simulink model "IEEE123_4subsystem"  (R2022b)
settings: Solver=ode4  StartTime=0.0  StopTime=inf  FixedStep=Ts  MaxStep=1e-4  RelTol=1e-3
PreLoadFcn:
  | Ts = 50e-6;
PostLoadFcn:
  | Ts = 50e-6;
InitFcn:
  | %%%%%%%%%%%%%%%%%%%%%%%%
  | % Simulation data for the IEEE 123 Node Test Feeder model
  | %%%%%%%%%%%%%%%%%%%%%%%
  | 
  | % miles/km
  | mi2km = 1.60934;
  | 
  | % feet to km
  | ft2km = 0.0003048;
  | 
  | % microsiemens to Farads
  | ms2F = 1/2/pi/60*1e-6;
  | 
  | %% Configuration 1 - series reactance - ohm/mile
  | 
  | R_1 = [0.4576 0.1560 0.1535;0.1560 0.4666 0.1580;0.1535 0.1580 0.4615];
  | X_1 = [1.0780 0.5017 0.3849;0.5017 1.0482 0.4236;0.3849 0.4236 1.0651];
  | 
  | % charging susceptance - microsiemens/mile
  | 
  | B_1 = [5.6765 -1.8319 -0.6982;-1.8319 5.9809 -1.1645;-0.6982 -1.1645 5.3971];
  | 
  | % convert for SPS
  | 
  | R_1 = R_1/mi2km;
  | 
  | Rs_1=(R_1(1,1)+R_1(2,2)+R_1(3,3))/3;
  | Rm_1=(R_1(1,2)+R_1(1,3)+R_1(2,3))/3;
  | R1_1=Rs_1-Rm_1;
  | R0_1=Rs_1+2*Rm_1;
  | 
  | L_1 = X_1/mi2km/2/pi/60;
  | 
  | Ls_1=(L_1(1,1)+L_1(2,2)+L_1(3,3))/3;
  | Lm_1=(L_1(1,2)+L_1(1,3)+L_1(2,3))/3;
  | L1_1=Ls_1-Lm_1;
  | L0_1=Ls_1+2*Lm_1;
  | 
  | C_1 = B_1/mi2km*ms2F;
  | 
  | Cs_1=(C_1(1,1)+C_1(2,2)+C_1(3,3))/3;
  | Cm_1=(C_1(1,2)+C_1(1,3)+C_1(2,3))/3;
  | C1_1=Cs_1-Cm_1;
  | C0_1=Cs_1+2*Cm_1;
  | 
  | 
  | %% Configuration 2 - series reactance - ohm/mile
  | 
  | R_2 = [0.4666 0.1580 0.1560;0.1580 0.4615 0.1535;0.1560 0.1535 0.4576];
  | X_2 = [1.0482 0.4236 0.5017;0.4236 1.0651 0.3849;0.5017 0.3849 1.0780];
  | 
  | % charging susceptance - microsiemens/mile
  | 
  | B_2 = [5.9809 -1.1645 -1.8319;-1.1645 5.3971 -0.6982;-1.8319 -0.6982 5.6765];
  | 
  | % convert for SPS
  | 
  | R_2 = R_2/mi2km;
  | 
  | Rs_2=(R_2(1,1)+R_2(2,2)+R_2(3,3))/3;
  | ... (+341 lines)
undefined symbols (not defined in the file): D1, Delta, find_system, I, Left, MOV_segment9, powergui, Right, type, V, X
libraries: spsGroundLib x242, spsThreePhaseVIMeasurementLib x134, spsSeriesRLCBranchLib x107, spsSeriesRLCLoadLib x83, spsPiSectionLineLib x61, spsThreePhasePISectionLineLib x60, spsVoltageMeasurementLib x52, spsDCVoltageSourceLib x36, ssn_lib x28, artemis x24, spsACCurrentSourceLib x18, spsOnDelayLib x18
(part 9 of 15)

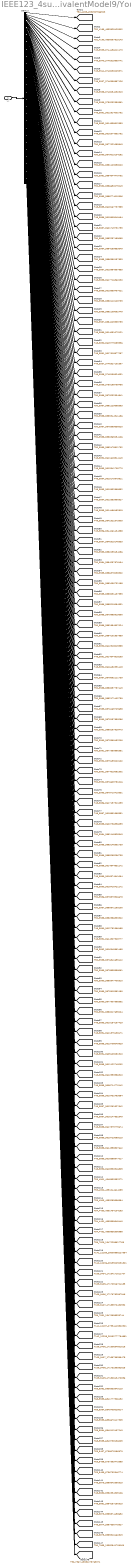
== system IEEE123_4subsystem/powergui/EquivalentModel9/Yout ==
  v,i : Inport
  Demux : Demux  Outputs=[1 1 1 1 1 1 1 1 1 1 1 1 1 1 1 1 1 1 1 1 1 1 1 1 1 1 1 1 1 1 1 1 1 1 1 1 1 1 1 1 1 1 1 1 1 1 1 1 1 1 1 1 1 1 1 1 1 1 1 1 1 1 1 1 1 1 1 1 1 1 1 1 1 1 1 1 1 1 1 1 1 1 1 1 1 1 1 1 1 1 1 1 1 1 1 1 1 1 1 1 1 1 1 1 1 1 1 1 1 1 1 1 1 1 1 1 1 1 1 1 1 1 1 1 1 1 1 1 1 1 1 1 1 1 1 1 1 1 1 1 1 1 1 1 1 1 1 1]
  tag scope: T109_9404_17164171611707=global, T109_9405_17170316724185=global, T109_9406_17160654601616=global, T109_9406_17176782997946=global, T109_9407_17166796396478=global, T109_9407_17183570432992=global, T109_9408_17173259352625=global, T109_9409_17180043470056=global, T141_12185_28000866227554=global, T141_12187_27994413822521=global, T142_12236_28199229231821=global, T142_12238_28192777784881=global, T48_3873_3585874458652=global, T48_3874_3587636775527=global, T48_3875_3589510462819=global, T48_3879_3580642690315=global, T48_3880_3582394305106=global, T48_3881_3584257290315=global, T48_3885_3618167737589=global, T48_3886_3617157911059=global, T48_3886_3619903049464=global, T48_3887_3615984597855=global, T48_3887_3616147832549=global, T48_3887_3618891568351=global, T48_3887_3621749731755=global, T48_3888_3614844831272=global, T48_3888_3614958807642=global, T48_3888_3617716362230=global, T48_3888_3617879775674=global, T48_3888_3620736596059=global, T48_3889_3614051073121=global, T48_3889_3616574941064=global, T48_3889_3616688977017=global, T48_3889_3619559497021=global, T48_3889_3619723089215=global, T48_3890_3612781366485=global, T48_3890_3612918015585=global, T48_3890_3615779289996=global, T48_3890_3618416421272=global, T48_3890_3618530516809=global, T48_3891_3612814002762=global, T48_3891_3614507928777=global, T48_3891_3614644518293=global, T48_3891_3617618877287=global, T48_3892_3611618814145=global, T48_3892_3614538612553=global, T48_3892_3616345861485=global, T48_3892_3616482391418=global, T48_3893_3610154197429=global, T48_3893_3610932868652=global, T48_3893_3613341709770=global, T48_3893_3616374592762=global, T48_3894_3609403281910=global, T48_3894_3611875438471=global, T48_3894_3612653990527=global, T48_3894_3615175975811=global, T48_3895_3608714770142=global, T48_3895_3611122749202=global, T48_3895_3613708049929=global, T48_3895_3614486482819=global, T48_3896_3610432463684=global, T48_3896_3612953586910=global, T48_3897_3612261527642=global, T49_3895_3842322373503=global, T49_3896_3844261434388=global, T49_3897_3846315148333=global, T49_3937_3746327101667=global, T49_3937_3746390887126=global, T49_3938_3748190624031=global, T49_3938_3748254292313=global, T49_3939_3744456211173=global, T49_3939_3750168799456=global, T49_3939_3750232350561=global, T49_3940_3746315893741=global, T49_3941_3748290229371=global, T50_3981_3884644479792=global, T50_3982_3886650275249=global, T50_3983_3882255454286=global, T50_3983_3882257489065=global, T50_3983_3888774010306=global, T50_3984_3881090731188=global, T50_3984_3881145828343=global, T50_3984_3884257876494=global, T50_3984_3884259853649=global, T50_3985_3879985915690=global, T50_3985_3880110128739=global, T50_3985_3883091437959=global, T50_3985_3883146592739=global, T50_3985_3886378238302=global, T50_3985_3886380157833=global, T50_3986_3878873926678=global, T50_3986_3879232334841=global, T50_3986_3881984907024=global, T50_3986_3882109062449=global, T50_3986_3885210084331=global, T50_3986_3885265296735=global, T50_3987_3878062111739=global, T50_3987_3878369636020=global, T50_3987_3880871260200=global, T50_3987_3881229668363=global, T50_3987_3884101837959=global, T50_3987_3884225935759=global, T50_3988_3876841655412=global, T50_3988_3880057787449=global, T50_3988_3880365254106=global, T50_3988_3882986533322=global, T50_3988_3883344941486=global, T50_3989_3875915381180=global, T50_3989_3876165729698=global, T50_3989_3877021089943=global, T50_3989_3878835558061=global, T50_3989_3882171402759=global, T50_3989_3882478811792=global, T50_3990_3875360452200=global, T50_3990_3877907568392=global, T50_3990_3878157859286=global, T50_3990_3879013104282=global, T50_3990_3880947400310=global, T50_3991_3874615082302=global, T50_3991_3877350866351=global, T50_3991_3880017695204=global, T50_3991_3880267928473=global, T50_3991_3881123058220=global, T50_3992_3876603781016=global, T50_3992_3879459220102=global, T50_3993_3878710419331=global, T52_4188_4531907566923=global, T52_4189_4533925429302=global, T52_4190_4536067815143=global, T53_4301_4348933352271=global, T53_4302_4351044614289=global, T53_4303_4353283696684=global, T54_4430_4591494104263=global, T54_4431_4593599645440=global, T54_4432_4595836306988=global, T63_5457_6798078186979=global, T63_5458_6797363473385=global, T63_5459_6796792546774=global, T68_5582_6838333543115=global, T68_5583_6836670417305=global, T68_5583_6841777506152=global, T68_5584_6840112497243=global, T68_5584_6845405028014=global, T68_5585_6843738136005=global, T89_7929_13472298617768=global, T89_7931_13470698333744=global, T90_7965_13382841709169=global, T90_7967_13381278763371=global
  wires:
  v,i/1 -> Demux/1
  Demux/1 -> [T52_4188_4531907566923]
  Demux/2 -> [T52_4189_4533925429302]
  Demux/3 -> [T52_4190_4536067815143]
  Demux/4 -> [T49_3939_3744456211173]
  Demux/5 -> [T49_3940_3746315893741]
  Demux/6 -> [T49_3941_3748290229371]
  Demux/7 -> [T49_3937_3746390887126]
  Demux/8 -> [T49_3938_3748254292313]
  Demux/9 -> [T49_3939_3750232350561]
  Demux/10 -> [T48_3891_3612814002762]
  Demux/11 -> [T48_3892_3614538612553]
  Demux/12 -> [T48_3893_3616374592762]
  Demux/13 -> [T50_3989_3877021089943]
  Demux/14 -> [T50_3990_3879013104282]
  Demux/15 -> [T50_3991_3881123058220]
  Demux/16 -> [T50_3981_3884644479792]
  Demux/17 -> [T50_3982_3886650275249]
  Demux/18 -> [T50_3983_3888774010306]
  Demux/19 -> [T48_3885_3618167737589]
  Demux/20 -> [T48_3886_3619903049464]
  Demux/21 -> [T48_3887_3621749731755]
  Demux/22 -> [T50_3983_3882257489065]
  Demux/23 -> [T50_3984_3884259853649]
  Demux/24 -> [T50_3985_3886380157833]
  Demux/25 -> [T48_3887_3615984597855]
  Demux/26 -> [T48_3888_3617716362230]
  Demux/27 -> [T48_3889_3619559497021]
  Demux/28 -> [T50_3985_3880110128739]
  Demux/29 -> [T50_3986_3882109062449]
  Demux/30 -> [T50_3987_3884225935759]
  Demux/31 -> [T48_3889_3614051073121]
  Demux/32 -> [T48_3890_3615779289996]
  Demux/33 -> [T48_3891_3617618877287]
  Demux/34 -> [T49_3937_3746327101667]
  Demux/35 -> [T49_3938_3748190624031]
  Demux/36 -> [T49_3939_3750168799456]
  Demux/37 -> [T50_3986_3879232334841]
  Demux/38 -> [T50_3987_3881229668363]
  Demux/39 -> [T50_3988_3883344941486]
  Demux/40 -> [T50_3987_3878369636020]
  Demux/41 -> [T50_3988_3880365254106]
  Demux/42 -> [T50_3989_3882478811792]
  Demux/43 -> [T48_3892_3611618814145]
  Demux/44 -> [T48_3893_3613341709770]
  Demux/45 -> [T48_3894_3615175975811]
  Demux/46 -> [T48_3893_3610932868652]
  Demux/47 -> [T48_3894_3612653990527]
  Demux/48 -> [T48_3895_3614486482819]
  Demux/49 -> [T49_3895_3842322373503]
  Demux/50 -> [T49_3896_3844261434388]
  Demux/51 -> [T49_3897_3846315148333]
  Demux/52 -> [T50_3983_3882255454286]
  Demux/53 -> [T50_3984_3884257876494]
  Demux/54 -> [T50_3985_3886378238302]
  Demux/55 -> [T50_3984_3881090731188]
  Demux/56 -> [T50_3985_3883091437959]
  Demux/57 -> [T50_3986_3885210084331]
  Demux/58 -> [T50_3985_3879985915690]
  Demux/59 -> [T50_3986_3881984907024]
  Demux/60 -> [T50_3987_3884101837959]
  Demux/61 -> [T48_3890_3612918015585]
  Demux/62 -> [T48_3891_3614644518293]
  Demux/63 -> [T48_3892_3616482391418]
  Demux/64 -> [T50_3987_3878062111739]
  Demux/65 -> [T50_3988_3880057787449]
  Demux/66 -> [T50_3989_3882171402759]
  Demux/67 -> [T50_3989_3876165729698]
  Demux/68 -> [T50_3990_3878157859286]
  Demux/69 -> [T50_3991_3880267928473]
  Demux/70 -> [T50_3990_3875360452200]
  Demux/71 -> [T50_3991_3877350866351]
  Demux/72 -> [T50_3992_3879459220102]
  Demux/73 -> [T50_3991_3874615082302]
  Demux/74 -> [T50_3992_3876603781016]
  Demux/75 -> [T50_3993_3878710419331]
  Demux/76 -> [T48_3886_3617157911059]
  Demux/77 -> [T48_3887_3618891568351]
  Demux/78 -> [T48_3888_3620736596059]
  Demux/79 -> [T50_3984_3881145828343]
  Demux/80 -> [T50_3985_3883146592739]
  Demux/81 -> [T50_3986_3885265296735]
  Demux/82 -> [T48_3888_3614844831272]
  Demux/83 -> [T48_3889_3616574941064]
  Demux/84 -> [T48_3890_3618416421272]
  Demux/85 -> [T50_3986_3878873926678]
  Demux/86 -> [T50_3987_3880871260200]
  Demux/87 -> [T50_3988_3882986533322]
  Demux/88 -> [T48_3890_3612781366485]
  Demux/89 -> [T48_3891_3614507928777]
  Demux/90 -> [T48_3892_3616345861485]
  Demux/91 -> [T50_3988_3876841655412]
  Demux/92 -> [T50_3989_3878835558061]
  Demux/93 -> [T50_3990_3880947400310]
  Demux/94 -> [T50_3989_3875915381180]
  Demux/95 -> [T50_3990_3877907568392]
  Demux/96 -> [T50_3991_3880017695204]
  Demux/97 -> [T48_3893_3610154197429]
  Demux/98 -> [T48_3894_3611875438471]
  Demux/99 -> [T48_3895_3613708049929]
  Demux/100 -> [T48_3894_3609403281910]
  Demux/101 -> [T48_3895_3611122749202]
  Demux/102 -> [T48_3896_3612953586910]
  Demux/103 -> [T48_3895_3608714770142]
  Demux/104 -> [T48_3896_3610432463684]
  Demux/105 -> [T48_3897_3612261527642]
  Demux/106 -> [T48_3887_3616147832549]
  Demux/107 -> [T48_3888_3617879775674]
  Demux/108 -> [T48_3889_3619723089215]
  Demux/109 -> [T48_3888_3614958807642]
  Demux/110 -> [T48_3889_3616688977017]
  Demux/111 -> [T48_3890_3618530516809]
  Demux/112 -> [T53_4301_4348933352271]
  Demux/113 -> [T53_4302_4351044614289]
  Demux/114 -> [T53_4303_4353283696684]
  Demux/115 -> [T54_4430_4591494104263]
  Demux/116 -> [T54_4431_4593599645440]
  Demux/117 -> [T54_4432_4595836306988]
  Demux/118 -> [T89_7929_13472298617768]
  Demux/119 -> [T141_12185_28000866227554]
  Demux/120 -> [T142_12236_28199229231821]
  Demux/121 -> [T109_9404_17164171611707]
  Demux/122 -> [T109_9405_17170316724185]
  Demux/123 -> [T109_9406_17176782997946]
  Demux/124 -> [T109_9407_17183570432992]
  Demux/125 -> [T89_7931_13470698333744]
  Demux/126 -> [T141_12187_27994413822521]
  Demux/127 -> [T142_12238_28192777784881]
  Demux/128 -> [T109_9406_17160654601616]
  Demux/129 -> [T109_9407_17166796396478]
  Demux/130 -> [T109_9408_17173259352625]
  Demux/131 -> [T109_9409_17180043470056]
  Demux/132 -> [T68_5582_6838333543115]
  Demux/133 -> [T68_5583_6841777506152]
  Demux/134 -> [T68_5584_6845405028014]
  Demux/135 -> [T68_5583_6836670417305]
  Demux/136 -> [T68_5584_6840112497243]
  Demux/137 -> [T68_5585_6843738136005]
  Demux/138 -> [T63_5457_6798078186979]
  Demux/139 -> [T63_5458_6797363473385]
  Demux/140 -> [T63_5459_6796792546774]
  Demux/141 -> [T48_3879_3580642690315]
  Demux/142 -> [T48_3880_3582394305106]
  Demux/143 -> [T48_3881_3584257290315]
  Demux/144 -> [T48_3873_3585874458652]
  Demux/145 -> [T48_3874_3587636775527]
  Demux/146 -> [T48_3875_3589510462819]
  Demux/147 -> [T90_7965_13382841709169]
  Demux/148 -> [T90_7967_13381278763371]

== system IEEE123_4subsystem/SM_123p/Regulator 1 Three Phase Ganged SVR/Single Phase SVR_A/Transformer with Taps ==
  note: Isec on CT Ratio base
  note: Vsec on Pt Ratio base
  N : Inport
  "   " : Terminator
  "    " : Gain  Gain=1/ptRatio
  " 1" : Gain  Gain=-1/ctRatio
  Back-Euler : Constant
  CT1 : spsCurrentMeasurementLib/Current Measurement  PhasorSimulation=off  OutputType=Complex  PSBequivalent=0
  Fcn : Fcn  Expr=1+0.1*u(1)/16
  Ground1 : spsGroundLib/Ground  LConnTagsString=a
  Memory : Memory
  Memory1 : Memory
  Mux1 : Mux  Inputs=2
  PT : spsVoltageMeasurementLib/Voltage Measurement  PhasorSimulation=off  OutputType=Complex  PSBequivalent=0
  SSN Interface Block (1ph) : ssn_lib/SSN Interface Block (1ph)  nb_phase=1  nb_port=2  p1_type=I-type(Left)  p2_type=X-type(Right)  p3_type=V-type(Left)  p4_type=V-type(Left)  p5_type=V-type(Left)  p6_type=V-type(Left)  p7_type=V-type(Left)  p8_type=V-type(Left)  p9_type=V-type(Left)  p10_type=V-type(Left)  p11_type=V-type(Left)  p12_type=V-type(Left)  p13_type=V-type(Left)  p14_type=V-type(Left)  p15_type=V-type(Left)  p16_type=V-type(Left)  I_port_shunt_resistance=1e9
  SSN Interface Block (1ph)2 : ssn_lib/SSN Interface Block (1ph)  nb_phase=1  nb_port=2  p1_type=X-type(Left)  p2_type=I-type(Right)  p3_type=X-type(Left)  p4_type=V-type (Right)  p5_type=V-type(Left)  p6_type=V-type(Left)  p7_type=V-type(Left)  p8_type=V-type(Left)  p9_type=V-type(Left)  p10_type=V-type(Left)  p11_type=V-type(Left)  p12_type=V-type(Left)  p13_type=V-type(Left)  p14_type=V-type(Left)  p15_type=V-type(Left)  p16_type=V-type(Left)  I_port_shunt_resistance=1e9
  SSN OLTC xfo v2 : Subsystem  AncestorBlock=artemis/SSN/SSN OLTC/SSN OLTC xfo v2  mask(Norton-Type External Nodal Subsystem){nnode=2, taggg=201x9172x689cf8bd979c, conntype=2 ports, RLpri=[1e-3 1e-4], Rcore=10000, ensat=off, Lcore=100, Lsat=1, phisat=100, Ts=Ts}
      mask prompts: nnode "Number of Electric nodes"; taggg "Unique Tag Identifier (automatic)"; conntype "Connection type"; RLpri "Primary winding resistance and inductance ([Ohms H])"; Rcore "Core Resistance (Ohms)"; ensat "Enable Saturation"; Lcore "Unsaturated magnetisation inductance (H)"; Lsat "Saturated magnetisation inductance (H)"; phisat "Flux saturation threshold (Weber)"; Ts "Sample Time (s)"
      mask help:
      | Continuously-variable On-Load Tapped Transformer (OLTC) (SSN Custom model)
      |
      | This block implements a 2 winding OLTC saturable transformer in SSN.
      | The model has a variable secondary inductance and resistance as well as turn-ratio.
      | The secondary winding is on the side marked with 'TAP'
      |
      | Mask parameters:
      |    Unique Tag Identifier: unique tag required by SSN to recknonize SSN external models
      |    Primary winding resistance and inductance ([Ohms H])
      |    Core Resistance (Ohms)
      |    Unsaturated magnetisation inductance (H): unsaturated core magnetization inductance
      |    Saturated magnetisation inductance (H): local inductance of the core in the saturated region
      |    Flux saturation threshold (Weber): flux saturation point
      |
      | Signal parameters:
      |
      | Signal inputs:
      |    1st sig: secondary winding resistance (Ohms)
      |    2nd sig: secondary winding inductance (H)
      |    3rd sig: transformer turn ratio k (V_secondary_tapped=k*V_primary)
      |    4th sig:  when set to 1, uses the Backward Euler method for solver. This can be used dynamically during simulation for example to damp numerical oscillations after switching events or after tap changes.
      |
      | Signals ouputs:
      |    1st signal: primary input current (A)
      |    2nd signal: secondary winding current (A)
      |    3rd signal: transformer flux (Wb)
      |
      | Saturation characteristic:
      |          flux
      |             ^              2
      |             |      1       *   <--- slope between point1 and point2 is Lsaturated
      |  phisat  |-----*  <---  this is the knee of flux=f(imag)
      |             |
      |             |
      |             |  <-----slope between origin and point1 is Lunsaturated
      |             *-------------------> imag
      mask init:
      | bloc=gcb;
      | taggg=get_param(bloc,'taggg');
      | conntyp=get_param(bloc,'conntype');
      | set_param([bloc '/FromV'],'GotoTag',['ssn_ext_sys_from_V_' taggg]);
      | set_param([bloc '/GotoHist'],'GotoTag',['ssn_ext_sys_goto_Hist_' taggg]);
      | set_param([bloc '/GotoY'],'GotoTag',['ssn_ext_sys_goto_Y_' taggg]);
      | 
      | R1=RLpri(1);
      | L1=RLpri(2);
      | 
      | if isequal(get_param(bloc,'ensat'),'off')
      |     phisat=1e20;
      | end
      | 
      | if isequal(conntyp,'4 ports')
      |     vin_sel=[1 2 3 4];
      |     Vinzeros=0;
      |     hist_sel=[1 2 3 4];
      |     a1=0;a2=0;a3=100;a4=100; b1=[7,34,40,33,31,33,40,33,31,33,40,33,31,33,40,34,7];b2=[30,30,34,42,40,37,45,52,50,47,54,62,59,57,65,70,70];b3=[93,67,60,67,70,67,60,67,70,67,60,67,70,67,60,67,93];b4=[30,30,34,42,40,37,45,52,50,47,54,62,60,57,65,70,70];
      |     c1=[20,20]*0;c2=[20,30]*0;c3=[27,14]*0;c4=[20,20]*0;c5=[24,17]*0;c6=[16,16]*0;c7=[22,19]*0;c8=[13,13]*0;c9=[80,80]*0;c10=[20,30]*0;c11=[88,74]*0;c12=[20,20]*0;c13=[85,77]*0;c14=[16,16]*0;c15=[81,79]*0;c16=[13,13]*0;
      |     %d1=[85,80];d2=[60,60];d3=[83,83];d4=[50,60];d5=[90,88,86];d6=[50,60,50];d7=[89,87];d8=[54,54];d9=[92,95,96,96,95,92,92];d10=[53,53,55,58,60,60,50];
      | 
      | 
      | elseif isequal(conntyp,'3 ports (primary grounded)')
      |     vin_sel=[1 2 5 3];
      |     Vinzeros=[0 0];
      |     hist_sel=[1 2 4];
      |   
      |      a1=0;a2=0;a3=100;a4=100; b1=[20,34,40,33,31,33,40,33,31,33,40,33,31,33,40,34,7];b2=[30,30,34,42,40,37,45,52,50,47,54,62,59,57,65,70,70];b3=[93,67,60,67,70,67,60,67,70,67,60,67,70,67,60,67,93];b4=[30,30,34,42,40,37,45,52,50,47,54,62,60,57,65,70,70];
      |     c1=[20,20];c2=[20,30];c3=[27,14];c4=[20,20];c5=[24,17];c6=[16,16];c7=[22,19];c8=[13,13];c9=[80,80]*0;c10=[20,30]*0;c11=[88,74]*0;c12=[20,20]*0;c13=[85,77]*0;c14=[16,16]*0;c15=[81,79]*0;c16=[13,13]*0;
      |     %d1=[85,80];d2=[60,60];d3=[83,83];d4=[50,60];d5=[90,88,86];d6=[50,60,50];d7=[89,87];d8=[54,54];d9=[92,95,96,96,95,92,92];d10=[53,53,55,58,60,60,50];
      | elseif isequal(conntyp,'3 ports (tapped secondary grounded)')
      |     vin_sel=[1 2 3 5];
      |     Vinzeros=[0 0];
      |     hist_sel=[1 2 3];
      |  
      |    a1=0;a2=0;a3=100;a4=100; b1=[20,34,40,33,31,33,40,33,31,33,40,33,31,33,40,34,7];b2=[30,30,34,42,40,37,45,52,50,47,54,62,59,57,65,70,70];b3=[80,67,60,67,70,67,60,67,70,67,60,67,70,67,60,67,93];b4=[30,30,34,42,40,37,45,52,50,47,54,62,60,57,65,70,70];
      |     c1=[20,20]*0;c2=[20,30]*0;c3=[27,14]*0;c4=[20,20]*0;c5=[24,17]*0;c6=[16,16]*0;c7=[22,19]*0;c8=[13,13]*0;c9=[80,80];c10=[20,30];c11=[88,74];c12=[20,20];c13=[85,77];c14=[16,16];c15=[81,79];c16=[13,13];
      |     %d1=[85,80];d2=[60,60];d3=[83,83];d4=[50,60];d5=[90,88,86];d6=[50,60,50];d7=[89,87];d8=[54,54];d9=[92,95,96,96,95,92,92];d10=[53,53,55,58,60,60,50];
      | elseif isequal(conntyp,'2 ports')
      |     vin_sel=[1 2 5 5];
      |     Vinzeros=[0 0 0];
      |     hist_sel=[1 2];
      |         a1=0;a2=0;a3=100;a4=100; b1=[20,34,40,33,31,33,40,33,31,33,40,33,31,33,40,34,7];b2=[30,30,34,42,40,37,45,52,50,47,54,62,59,57,65,70,70];b3=[80,67,60,67,70,67,60,67,70,67,60,67,70,67,60,67,93];b4=[30,30,34,42,40,37,45,52,50,47,54,62,60,57,65,70,70];
      |     c1=[20,20];c2=[20,30];c3=[27,14];c4=[20,20];c5=[24,17];c6=[16,16];c7=[22,19];c8=[13,13];c9=[80,80];c10=[20,30];c11=[88,74];c12=[20,20];c13=[85,77];c14=[16,16];c15=[81,79];c16=[13,13];
      |     %d1=[85,80];d2=[60,60];d3=[83,83];d4=[50,60];d5=[90,88,86];d6=[50,60,50];d7=[89,87];d8=[54,54];d9=[92,95,96,96,95,92,92];d10=[53,53,55,58,60,60,50];
      | else
      | 
      | end
      | 
      | ori=get_param(bloc,'Orientation');
      | 
      | if isequal(ori,'right')
      |     d1=[73,67];d2=[56,56];d3=[70,70];d4=[45,56];d5=[80,77,75];d6=[45,56,45];d7=[79,76];d8=[50,50];d9=[82,84,86,84,82,82];d10=[50,50,54,56,56,45];
      | else
      |     d1=[73,71,69,71,73,73];d2=[50,50,52,56,56,45];d3=[80,77,75];d4=[45,56,45];d5=[76,79];d6=[50,50];d7=[88,82];d8=[56,56];d9=[85,85];d10=[45,56];
      | end
      settings: LibrarySourceBlock=artemis/SSN/SSN OLTC/SSN OLTC xfo v2
      settings: CopyFcn=|
      | str=tempname;
      | str=strrep(str(end-20:end),'_','x');
      | set_param(gcb,'taggg',str);
      | set_param(gcb,'LinkStatus','inactive');
      mask Help: eval('open SSN_OLTC.pdf;');
      mask TypeOptions conntype: 4 ports | 3 ports (primary grounded) | 3 ports (tapped secondary grounded) | 2 ports
      mask Callback conntype:
      | bloc=gcb;
      | conntyp=get_param(bloc,'conntype');
      | nn=fts6_xfo_port_cb(bloc,conntyp);
      | set_param(bloc,'nnode',nn);
      mask Display:
      | plot(a1,a2,a3,a4,b1,b2,b3,b4,c1,c2,c3,c4,c5,c6,c7,c8,c9,c10,c11,c12,c13,c14,c15,c16);
      | color('blue');
      | plot(d1,d2,d3,d4,d5,d6,d7,d8,d9,d10);
  Transfo R2-L2-turnratio : Constant  Value=[0.0001 0.00001 1]
  x : Product  RndMeth=Zero
  L : PMIOPort  Tag=PMCPort  Side=Right
  S : PMIOPort  Port=2  Side=Left
  Isec : Outport
  Vsec : Outport  Port=2
  wires:
  Memory/1 -> Isec/1
  Memory1/1 -> Vsec/1
  " 1"/1 -> Memory/1
  CT1/1 -> " 1"/1
  PT/1 -> "    "/1
  "    "/1 -> Memory1/1
  N/1 -> Fcn/1
  SSN OLTC xfo v2/1(meas) -> "   "/1  "transfo flux (Weber)"
  Back-Euler/1 -> Mux1/2
  Transfo R2-L2-turnratio/1 -> x/2
  x/1 -> Mux1/1
  Mux1/1 -> SSN OLTC xfo v2/1(params)
  Fcn/1 -> x/1
  connections:
  CT1/LConn1 -- L/RConn1
  PT/LConn2 -- Ground1/LConn1
  S/RConn1 -- SSN Interface Block (1ph)/LConn1
  SSN OLTC xfo v2/RConn1 -- SSN Interface Block (1ph)2/LConn1
  SSN OLTC xfo v2/LConn1 -- SSN Interface Block (1ph)/RConn1
  SSN Interface Block (1ph)2/RConn1 -- CT1/RConn1 -- PT/LConn1

== system IEEE123_4subsystem/SM_123p/Regulator 1 Three Phase Ganged SVR/Single Phase SVR_A/Voltage Regulator Control ==
  Vm : Inport
  Constant : Constant  Value=RegulatorOn
  Tap Changer Control : Subsystem  mask(Tap Changer Control){MinMaxTap=TapMinMax, InitialPosition=InitialTap, MecDelay=TapSelectionTime}
      mask prompts: MinMaxTap "Minimum and maximum tap number [ Min  Max ] :"; InitialPosition "Initial tap position"; MecDelay "Mechanical delay time"
      mask init:
      | if MecDelay<=0,
      | 	MecDelay=1/60;
      | end
  Voltage regulator : Subsystem  mask{Vref=RegulatorVref*120, DeadBand=RegulatorDeadBand*120, TimeDelay=RegulatorDelay}
      mask prompts: Vref "Vref (on 120v base)"; DeadBand "Deadband (on 120v base)"; TimeDelay "Time delay (s)"
  N : Outport
  Tap : Outport  Port=2
  wires:
  Vm/1 -> Voltage regulator/1(Vmes (pu))
  Constant/1 -> Voltage regulator/3(RegOn)
  Tap Changer Control/2(Ready) -> Voltage regulator/2(Ready)
  Voltage regulator/1(Up) -> Tap Changer Control/1("Up ")
  Tap Changer Control/1(TapNo) -> N/1, Tap/1  "Tap"
  Voltage regulator/2(Down) -> Tap Changer Control/2("Down ")

== system IEEE123_4subsystem/SM_123p/Regulator 1 Three Phase Ganged SVR/Single Phase SVR_B/Transformer with Taps ==
  note: Isec on CT Ratio base
  note: Vsec on Pt Ratio base
  N : Inport
  "   " : Terminator
  "    " : Gain  Gain=1/ptRatio
  " 1" : Gain  Gain=-1/ctRatio
  Back-Euler : Constant
  CT1 : spsCurrentMeasurementLib/Current Measurement  PhasorSimulation=off  OutputType=Complex  PSBequivalent=0
  Fcn : Fcn  Expr=1+0.1*u(1)/16
  Ground1 : spsGroundLib/Ground  LConnTagsString=a
  Memory : Memory
  Memory1 : Memory
  Mux1 : Mux  Inputs=2
  PT : spsVoltageMeasurementLib/Voltage Measurement  PhasorSimulation=off  OutputType=Complex  PSBequivalent=0
  SSN Interface Block (1ph) : ssn_lib/SSN Interface Block (1ph)  nb_phase=1  nb_port=2  p1_type=I-type(Left)  p2_type=X-type(Right)  p3_type=V-type(Left)  p4_type=V-type(Left)  p5_type=V-type(Left)  p6_type=V-type(Left)  p7_type=V-type(Left)  p8_type=V-type(Left)  p9_type=V-type(Left)  p10_type=V-type(Left)  p11_type=V-type(Left)  p12_type=V-type(Left)  p13_type=V-type(Left)  p14_type=V-type(Left)  p15_type=V-type(Left)  p16_type=V-type(Left)  I_port_shunt_resistance=1e9
  SSN Interface Block (1ph)2 : ssn_lib/SSN Interface Block (1ph)  nb_phase=1  nb_port=2  p1_type=X-type(Left)  p2_type=I-type(Right)  p3_type=X-type(Left)  p4_type=V-type (Right)  p5_type=V-type(Left)  p6_type=V-type(Left)  p7_type=V-type(Left)  p8_type=V-type(Left)  p9_type=V-type(Left)  p10_type=V-type(Left)  p11_type=V-type(Left)  p12_type=V-type(Left)  p13_type=V-type(Left)  p14_type=V-type(Left)  p15_type=V-type(Left)  p16_type=V-type(Left)  I_port_shunt_resistance=1e9
  SSN OLTC xfo v2 : Subsystem  AncestorBlock=artemis/SSN/SSN OLTC/SSN OLTC xfo v2  mask(Norton-Type External Nodal Subsystem){nnode=2, taggg=987xa5e3xeb9000d249b6, conntype=2 ports, RLpri=[1e-3 1e-4], Rcore=10000, ensat=off, Lcore=100, Lsat=1, phisat=100, Ts=Ts}
      mask prompts: nnode "Number of Electric nodes"; taggg "Unique Tag Identifier (automatic)"; conntype "Connection type"; RLpri "Primary winding resistance and inductance ([Ohms H])"; Rcore "Core Resistance (Ohms)"; ensat "Enable Saturation"; Lcore "Unsaturated magnetisation inductance (H)"; Lsat "Saturated magnetisation inductance (H)"; phisat "Flux saturation threshold (Weber)"; Ts "Sample Time (s)"
      mask help:
      | Continuously-variable On-Load Tapped Transformer (OLTC) (SSN Custom model)
      |
      | This block implements a 2 winding OLTC saturable transformer in SSN.
      | The model has a variable secondary inductance and resistance as well as turn-ratio.
      | The secondary winding is on the side marked with 'TAP'
      |
      | Mask parameters:
      |    Unique Tag Identifier: unique tag required by SSN to recknonize SSN external models
      |    Primary winding resistance and inductance ([Ohms H])
      |    Core Resistance (Ohms)
      |    Unsaturated magnetisation inductance (H): unsaturated core magnetization inductance
      |    Saturated magnetisation inductance (H): local inductance of the core in the saturated region
      |    Flux saturation threshold (Weber): flux saturation point
      |
      | Signal parameters:
      |
      | Signal inputs:
      |    1st sig: secondary winding resistance (Ohms)
      |    2nd sig: secondary winding inductance (H)
      |    3rd sig: transformer turn ratio k (V_secondary_tapped=k*V_primary)
      |    4th sig:  when set to 1, uses the Backward Euler method for solver. This can be used dynamically during simulation for example to damp numerical oscillations after switching events or after tap changes.
      |
      | Signals ouputs:
      |    1st signal: primary input current (A)
      |    2nd signal: secondary winding current (A)
      |    3rd signal: transformer flux (Wb)
      |
      | Saturation characteristic:
      |          flux
      |             ^              2
      |             |      1       *   <--- slope between point1 and point2 is Lsaturated
      |  phisat  |-----*  <---  this is the knee of flux=f(imag)
      |             |
      |             |
      |             |  <-----slope between origin and point1 is Lunsaturated
      |             *-------------------> imag
      mask init: same as IEEE123_4subsystem/SM_123p/Regulator 1 Three Phase Ganged SVR/Single Phase SVR_A/Transformer with Taps/SSN OLTC xfo v2
      settings: LibrarySourceBlock=artemis/SSN/SSN OLTC/SSN OLTC xfo v2
      settings: CopyFcn=|
      | str=tempname;
      | str=strrep(str(end-20:end),'_','x');
      | set_param(gcb,'taggg',str);
      | set_param(gcb,'LinkStatus','inactive');
      mask Help: eval('open SSN_OLTC.pdf;');
      mask TypeOptions conntype: 4 ports | 3 ports (primary grounded) | 3 ports (tapped secondary grounded) | 2 ports
      mask Callback conntype:
      | bloc=gcb;
      | conntyp=get_param(bloc,'conntype');
      | nn=fts6_xfo_port_cb(bloc,conntyp);
      | set_param(bloc,'nnode',nn);
      mask Display:
      | plot(a1,a2,a3,a4,b1,b2,b3,b4,c1,c2,c3,c4,c5,c6,c7,c8,c9,c10,c11,c12,c13,c14,c15,c16);
      | color('blue');
      | plot(d1,d2,d3,d4,d5,d6,d7,d8,d9,d10);
  Transfo R2-L2-turnratio : Constant  Value=[0.0001 0.00001 1]
  x : Product  RndMeth=Zero
  L : PMIOPort  Tag=PMCPort  Side=Right
  S : PMIOPort  Port=2  Side=Left
  Isec : Outport
  Vsec : Outport  Port=2
  wires:
  Memory/1 -> Isec/1
  Memory1/1 -> Vsec/1
  " 1"/1 -> Memory/1
  CT1/1 -> " 1"/1
  PT/1 -> "    "/1
  "    "/1 -> Memory1/1
  N/1 -> Fcn/1
  SSN OLTC xfo v2/1(meas) -> "   "/1  "transfo flux (Weber)"
  Back-Euler/1 -> Mux1/2
  Transfo R2-L2-turnratio/1 -> x/2
  x/1 -> Mux1/1
  Mux1/1 -> SSN OLTC xfo v2/1(params)
  Fcn/1 -> x/1
  connections:
  CT1/LConn1 -- L/RConn1
  PT/LConn2 -- Ground1/LConn1
  S/RConn1 -- SSN Interface Block (1ph)/LConn1
  SSN OLTC xfo v2/RConn1 -- SSN Interface Block (1ph)2/LConn1
  SSN OLTC xfo v2/LConn1 -- SSN Interface Block (1ph)/RConn1
  SSN Interface Block (1ph)2/RConn1 -- CT1/RConn1 -- PT/LConn1

== system IEEE123_4subsystem/SM_123p/Regulator 1 Three Phase Ganged SVR/Single Phase SVR_B/Voltage Regulator Control ==
  Vm : Inport
  Constant : Constant  Value=RegulatorOn
  Tap Changer Control : Subsystem  mask(Tap Changer Control){MinMaxTap=TapMinMax, InitialPosition=InitialTap, MecDelay=TapSelectionTime}
      mask prompts: MinMaxTap "Minimum and maximum tap number [ Min  Max ] :"; InitialPosition "Initial tap position"; MecDelay "Mechanical delay time"
      mask init:
      | if MecDelay<=0,
      | 	MecDelay=1/60;
      | end
  Voltage regulator : Subsystem  mask{Vref=RegulatorVref*120, DeadBand=RegulatorDeadBand*120, TimeDelay=RegulatorDelay}
      mask prompts: Vref "Vref (on 120v base)"; DeadBand "Deadband (on 120v base)"; TimeDelay "Time delay (s)"
  N : Outport
  Tap : Outport  Port=2
  wires:
  Vm/1 -> Voltage regulator/1(Vmes (pu))
  Constant/1 -> Voltage regulator/3(RegOn)
  Tap Changer Control/2(Ready) -> Voltage regulator/2(Ready)
  Voltage regulator/1(Up) -> Tap Changer Control/1("Up ")
  Tap Changer Control/1(TapNo) -> N/1, Tap/1  "Tap"
  Voltage regulator/2(Down) -> Tap Changer Control/2("Down ")

== system IEEE123_4subsystem/SM_123p/Regulator 1 Three Phase Ganged SVR/Single Phase SVR_C/Transformer with Taps ==
  note: Isec on CT Ratio base
  note: Vsec on Pt Ratio base
  N : Inport
  "   " : Terminator
  "    " : Gain  Gain=1/ptRatio
  " 1" : Gain  Gain=-1/ctRatio
  Back-Euler : Constant
  CT1 : spsCurrentMeasurementLib/Current Measurement  PhasorSimulation=off  OutputType=Complex  PSBequivalent=0
  Fcn : Fcn  Expr=1+0.1*u(1)/16
  Ground1 : spsGroundLib/Ground  LConnTagsString=a
  Memory : Memory
  Memory1 : Memory
  Mux1 : Mux  Inputs=2
  PT : spsVoltageMeasurementLib/Voltage Measurement  PhasorSimulation=off  OutputType=Complex  PSBequivalent=0
  SSN Interface Block (1ph) : ssn_lib/SSN Interface Block (1ph)  nb_phase=1  nb_port=2  p1_type=I-type(Left)  p2_type=X-type(Right)  p3_type=V-type(Left)  p4_type=V-type(Left)  p5_type=V-type(Left)  p6_type=V-type(Left)  p7_type=V-type(Left)  p8_type=V-type(Left)  p9_type=V-type(Left)  p10_type=V-type(Left)  p11_type=V-type(Left)  p12_type=V-type(Left)  p13_type=V-type(Left)  p14_type=V-type(Left)  p15_type=V-type(Left)  p16_type=V-type(Left)  I_port_shunt_resistance=1e9
  SSN Interface Block (1ph)2 : ssn_lib/SSN Interface Block (1ph)  nb_phase=1  nb_port=2  p1_type=X-type(Left)  p2_type=I-type(Right)  p3_type=X-type(Left)  p4_type=V-type (Right)  p5_type=V-type(Left)  p6_type=V-type(Left)  p7_type=V-type(Left)  p8_type=V-type(Left)  p9_type=V-type(Left)  p10_type=V-type(Left)  p11_type=V-type(Left)  p12_type=V-type(Left)  p13_type=V-type(Left)  p14_type=V-type(Left)  p15_type=V-type(Left)  p16_type=V-type(Left)  I_port_shunt_resistance=1e9
  SSN OLTC xfo v2 : Subsystem  AncestorBlock=artemis/SSN/SSN OLTC/SSN OLTC xfo v2  mask(Norton-Type External Nodal Subsystem){nnode=2, taggg=e52xa76ex313cf843a804, conntype=2 ports, RLpri=[1e-3 1e-4], Rcore=10000, ensat=off, Lcore=100, Lsat=1, phisat=100, Ts=Ts}
      mask prompts: nnode "Number of Electric nodes"; taggg "Unique Tag Identifier (automatic)"; conntype "Connection type"; RLpri "Primary winding resistance and inductance ([Ohms H])"; Rcore "Core Resistance (Ohms)"; ensat "Enable Saturation"; Lcore "Unsaturated magnetisation inductance (H)"; Lsat "Saturated magnetisation inductance (H)"; phisat "Flux saturation threshold (Weber)"; Ts "Sample Time (s)"
      mask help:
      | Continuously-variable On-Load Tapped Transformer (OLTC) (SSN Custom model)
      |
      | This block implements a 2 winding OLTC saturable transformer in SSN.
      | The model has a variable secondary inductance and resistance as well as turn-ratio.
      | The secondary winding is on the side marked with 'TAP'
      |
      | Mask parameters:
      |    Unique Tag Identifier: unique tag required by SSN to recknonize SSN external models
      |    Primary winding resistance and inductance ([Ohms H])
      |    Core Resistance (Ohms)
      |    Unsaturated magnetisation inductance (H): unsaturated core magnetization inductance
      |    Saturated magnetisation inductance (H): local inductance of the core in the saturated region
      |    Flux saturation threshold (Weber): flux saturation point
      |
      | Signal parameters:
      |
      | Signal inputs:
      |    1st sig: secondary winding resistance (Ohms)
      |    2nd sig: secondary winding inductance (H)
      |    3rd sig: transformer turn ratio k (V_secondary_tapped=k*V_primary)
      |    4th sig:  when set to 1, uses the Backward Euler method for solver. This can be used dynamically during simulation for example to damp numerical oscillations after switching events or after tap changes.
      |
      | Signals ouputs:
      |    1st signal: primary input current (A)
      |    2nd signal: secondary winding current (A)
      |    3rd signal: transformer flux (Wb)
      |
      | Saturation characteristic:
      |          flux
      |             ^              2
      |             |      1       *   <--- slope between point1 and point2 is Lsaturated
      |  phisat  |-----*  <---  this is the knee of flux=f(imag)
      |             |
      |             |
      |             |  <-----slope between origin and point1 is Lunsaturated
      |             *-------------------> imag
      mask init: same as IEEE123_4subsystem/SM_123p/Regulator 1 Three Phase Ganged SVR/Single Phase SVR_A/Transformer with Taps/SSN OLTC xfo v2
      settings: LibrarySourceBlock=artemis/SSN/SSN OLTC/SSN OLTC xfo v2
      settings: CopyFcn=|
      | str=tempname;
      | str=strrep(str(end-20:end),'_','x');
      | set_param(gcb,'taggg',str);
      | set_param(gcb,'LinkStatus','inactive');
      mask Help: eval('open SSN_OLTC.pdf;');
      mask TypeOptions conntype: 4 ports | 3 ports (primary grounded) | 3 ports (tapped secondary grounded) | 2 ports
      mask Callback conntype:
      | bloc=gcb;
      | conntyp=get_param(bloc,'conntype');
      | nn=fts6_xfo_port_cb(bloc,conntyp);
      | set_param(bloc,'nnode',nn);
      mask Display:
      | plot(a1,a2,a3,a4,b1,b2,b3,b4,c1,c2,c3,c4,c5,c6,c7,c8,c9,c10,c11,c12,c13,c14,c15,c16);
      | color('blue');
      | plot(d1,d2,d3,d4,d5,d6,d7,d8,d9,d10);
  Transfo R2-L2-turnratio : Constant  Value=[0.0001 0.00001 1]
  x : Product  RndMeth=Zero
  L : PMIOPort  Tag=PMCPort  Side=Right
  S : PMIOPort  Port=2  Side=Left
  Isec : Outport
  Vsec : Outport  Port=2
  wires:
  Memory/1 -> Isec/1
  Memory1/1 -> Vsec/1
  " 1"/1 -> Memory/1
  CT1/1 -> " 1"/1
  PT/1 -> "    "/1
  "    "/1 -> Memory1/1
  N/1 -> Fcn/1
  SSN OLTC xfo v2/1(meas) -> "   "/1  "transfo flux (Weber)"
  Back-Euler/1 -> Mux1/2
  Transfo R2-L2-turnratio/1 -> x/2
  x/1 -> Mux1/1
  Mux1/1 -> SSN OLTC xfo v2/1(params)
  Fcn/1 -> x/1
  connections:
  CT1/LConn1 -- L/RConn1
  PT/LConn2 -- Ground1/LConn1
  S/RConn1 -- SSN Interface Block (1ph)/LConn1
  SSN OLTC xfo v2/RConn1 -- SSN Interface Block (1ph)2/LConn1
  SSN OLTC xfo v2/LConn1 -- SSN Interface Block (1ph)/RConn1
  SSN Interface Block (1ph)2/RConn1 -- CT1/RConn1 -- PT/LConn1

== system IEEE123_4subsystem/SM_123p/Regulator 1 Three Phase Ganged SVR/Single Phase SVR_C/Voltage Regulator Control ==
  Vm : Inport
  Constant : Constant  Value=RegulatorOn
  Tap Changer Control : Subsystem  mask(Tap Changer Control){MinMaxTap=TapMinMax, InitialPosition=InitialTap, MecDelay=TapSelectionTime}
      mask prompts: MinMaxTap "Minimum and maximum tap number [ Min  Max ] :"; InitialPosition "Initial tap position"; MecDelay "Mechanical delay time"
      mask init:
      | if MecDelay<=0,
      | 	MecDelay=1/60;
      | end
  Voltage regulator : Subsystem  mask{Vref=RegulatorVref*120, DeadBand=RegulatorDeadBand*120, TimeDelay=RegulatorDelay}
      mask prompts: Vref "Vref (on 120v base)"; DeadBand "Deadband (on 120v base)"; TimeDelay "Time delay (s)"
  N : Outport
  Tap : Outport  Port=2
  wires:
  Vm/1 -> Voltage regulator/1(Vmes (pu))
  Constant/1 -> Voltage regulator/3(RegOn)
  Tap Changer Control/2(Ready) -> Voltage regulator/2(Ready)
  Voltage regulator/1(Up) -> Tap Changer Control/1("Up ")
  Tap Changer Control/1(TapNo) -> N/1, Tap/1  "Tap"
  Voltage regulator/2(Down) -> Tap Changer Control/2("Down ")

== system IEEE123_4subsystem/SM_123p/Regulator 2/Single Phase SVR_A/Line Drop Compensator ==
  note: Vm=Vsec-Isec(Rc+jXc)
  Isec : Inport
  Vsec : Inport  Port=2
  "        " : spsLinearTransformerLib/Linear Transformer  UNITS=SI  NominalPower=[pNom fNom]  winding1=[vNom/ptRatio 1e-7 1e-8]  winding2=[vNom/ptRatio 1e-7 1e-8]  ThreeWindings=off  winding3=[3.15e+005 0.7938 0.084225]  RmLm=[1e5 1e5]  Measurements=None  DataType=on
  "CTS  " : spsControlledCurrentSourceLib/Controlled Current Source  Initialize=on  Source_Type=AC  Amplitude=0  Phase=0  Frequency=0  Measurements=None
  "PTS  " : spsControlledVoltageSourceLib/Controlled Voltage Source  Initialize=on  Source_Type=AC  Amplitude=0  Phase=0  Frequency=0  Measurements=None
  RMS : spsRMSLib/RMS  TrueRMS=on  Freq=60  RMSInit=120  Ts=0
  Raux : spsSeriesRLCBranchLib/Series RLC Branch  LConnTagsString=__new0  RConnTagsString=__new0  BranchType=R  Resistance=1e3  Inductance=1.6 / (120*pi)  SetiL0=off  InitialCurrent=0  Capacitance=1e-6  Setx0=off  InitialVoltage=0  Measurements=None
  Rc+jXc : spsSeriesRLCBranchLib/Series RLC Branch  LConnTagsString=__new0  RConnTagsString=__new0  BranchType=RL  Resistance=Rc  Inductance=Xc / (2*pi*fNom)  SetiL0=off  InitialCurrent=0  Capacitance=1e-6  Setx0=off  InitialVoltage=0  Measurements=None
  VRelay : spsVoltageMeasurementLib/Voltage Measurement  PhasorSimulation=off  OutputType=Complex  PSBequivalent=0
  Vm : Outport
  wires:
  RMS/1 -> Vm/1
  VRelay/1 -> RMS/1
  Isec/1 -> "CTS  "/1
  Vsec/1 -> "PTS  "/1
  connections:
  "PTS  "/RConn1 -- "        "/RConn1
  "        "/RConn2 -- VRelay/LConn1
  Raux/LConn1 -- Rc+jXc/LConn1 -- "        "/LConn1 -- "CTS  "/RConn1
  Rc+jXc/RConn1 -- Raux/RConn1 -- "CTS  "/LConn1 -- "        "/LConn2
  VRelay/LConn2 -- "PTS  "/LConn1

== system IEEE123_4subsystem/SM_123p/Regulator 2/Single Phase SVR_A/Transformer with Taps ==
  note: Isec on CT Ratio base
  note: Vsec on Pt Ratio base
  N : Inport
  "   " : Terminator
  "    " : Gain  Gain=1/ptRatio
  " 1" : Gain  Gain=-1/ctRatio
  Back-Euler : Constant
  CT1 : spsCurrentMeasurementLib/Current Measurement  PhasorSimulation=off  OutputType=Complex  PSBequivalent=0
  Fcn : Fcn  Expr=1+0.1*u(1)/16
  Ground1 : spsGroundLib/Ground  LConnTagsString=a
  Memory : Memory
  Memory1 : Memory
  Mux1 : Mux  Inputs=2
  PT : spsVoltageMeasurementLib/Voltage Measurement  PhasorSimulation=off  OutputType=Complex  PSBequivalent=0
  SSN Interface Block (1ph) : ssn_lib/SSN Interface Block (1ph)  nb_phase=1  nb_port=2  p1_type=I-type(Left)  p2_type=X-type(Right)  p3_type=V-type(Left)  p4_type=V-type(Left)  p5_type=V-type(Left)  p6_type=V-type(Left)  p7_type=V-type(Left)  p8_type=V-type(Left)  p9_type=V-type(Left)  p10_type=V-type(Left)  p11_type=V-type(Left)  p12_type=V-type(Left)  p13_type=V-type(Left)  p14_type=V-type(Left)  p15_type=V-type(Left)  p16_type=V-type(Left)  I_port_shunt_resistance=1e9
  SSN Interface Block (1ph)2 : ssn_lib/SSN Interface Block (1ph)  nb_phase=1  nb_port=2  p1_type=X-type(Left)  p2_type=I-type(Right)  p3_type=X-type(Left)  p4_type=V-type (Right)  p5_type=V-type(Left)  p6_type=V-type(Left)  p7_type=V-type(Left)  p8_type=V-type(Left)  p9_type=V-type(Left)  p10_type=V-type(Left)  p11_type=V-type(Left)  p12_type=V-type(Left)  p13_type=V-type(Left)  p14_type=V-type(Left)  p15_type=V-type(Left)  p16_type=V-type(Left)  I_port_shunt_resistance=1e9
  SSN OLTC xfo v2 : Subsystem  AncestorBlock=artemis/SSN/SSN OLTC/SSN OLTC xfo v2  mask(Norton-Type External Nodal Subsystem){nnode=2, taggg=89bxbdb6x1398f6ae2864, conntype=2 ports, RLpri=[1e-3 1e-4], Rcore=10000, ensat=off, Lcore=100, Lsat=1, phisat=100, Ts=Ts}
      mask prompts: nnode "Number of Electric nodes"; taggg "Unique Tag Identifier (automatic)"; conntype "Connection type"; RLpri "Primary winding resistance and inductance ([Ohms H])"; Rcore "Core Resistance (Ohms)"; ensat "Enable Saturation"; Lcore "Unsaturated magnetisation inductance (H)"; Lsat "Saturated magnetisation inductance (H)"; phisat "Flux saturation threshold (Weber)"; Ts "Sample Time (s)"
      mask help:
      | Continuously-variable On-Load Tapped Transformer (OLTC) (SSN Custom model)
      |
      | This block implements a 2 winding OLTC saturable transformer in SSN.
      | The model has a variable secondary inductance and resistance as well as turn-ratio.
      | The secondary winding is on the side marked with 'TAP'
      |
      | Mask parameters:
      |    Unique Tag Identifier: unique tag required by SSN to recknonize SSN external models
      |    Primary winding resistance and inductance ([Ohms H])
      |    Core Resistance (Ohms)
      |    Unsaturated magnetisation inductance (H): unsaturated core magnetization inductance
      |    Saturated magnetisation inductance (H): local inductance of the core in the saturated region
      |    Flux saturation threshold (Weber): flux saturation point
      |
      | Signal parameters:
      |
      | Signal inputs:
      |    1st sig: secondary winding resistance (Ohms)
      |    2nd sig: secondary winding inductance (H)
      |    3rd sig: transformer turn ratio k (V_secondary_tapped=k*V_primary)
      |    4th sig:  when set to 1, uses the Backward Euler method for solver. This can be used dynamically during simulation for example to damp numerical oscillations after switching events or after tap changes.
      |
      | Signals ouputs:
      |    1st signal: primary input current (A)
      |    2nd signal: secondary winding current (A)
      |    3rd signal: transformer flux (Wb)
      |
      | Saturation characteristic:
      |          flux
      |             ^              2
      |             |      1       *   <--- slope between point1 and point2 is Lsaturated
      |  phisat  |-----*  <---  this is the knee of flux=f(imag)
      |             |
      |             |
      |             |  <-----slope between origin and point1 is Lunsaturated
      |             *-------------------> imag
      mask init: same as IEEE123_4subsystem/SM_123p/Regulator 1 Three Phase Ganged SVR/Single Phase SVR_A/Transformer with Taps/SSN OLTC xfo v2
      settings: LibrarySourceBlock=artemis/SSN/SSN OLTC/SSN OLTC xfo v2
      settings: CopyFcn=|
      | str=tempname;
      | str=strrep(str(end-20:end),'_','x');
      | set_param(gcb,'taggg',str);
      | set_param(gcb,'LinkStatus','inactive');
      mask Help: eval('open SSN_OLTC.pdf;');
      mask TypeOptions conntype: 4 ports | 3 ports (primary grounded) | 3 ports (tapped secondary grounded) | 2 ports
      mask Callback conntype:
      | bloc=gcb;
      | conntyp=get_param(bloc,'conntype');
      | nn=fts6_xfo_port_cb(bloc,conntyp);
      | set_param(bloc,'nnode',nn);
      mask Display:
      | plot(a1,a2,a3,a4,b1,b2,b3,b4,c1,c2,c3,c4,c5,c6,c7,c8,c9,c10,c11,c12,c13,c14,c15,c16);
      | color('blue');
      | plot(d1,d2,d3,d4,d5,d6,d7,d8,d9,d10);
  Transfo R2-L2-turnratio : Constant  Value=[0.0001 0.00001 1]
  x : Product  RndMeth=Zero
  L : PMIOPort  Tag=PMCPort  Side=Right
  S : PMIOPort  Port=2  Side=Left
  Isec : Outport
  Vsec : Outport  Port=2
  wires:
  Memory/1 -> Isec/1
  Memory1/1 -> Vsec/1
  " 1"/1 -> Memory/1
  CT1/1 -> " 1"/1
  PT/1 -> "    "/1
  "    "/1 -> Memory1/1
  N/1 -> Fcn/1
  SSN OLTC xfo v2/1(meas) -> "   "/1  "transfo flux (Weber)"
  Back-Euler/1 -> Mux1/2
  Transfo R2-L2-turnratio/1 -> x/2
  x/1 -> Mux1/1
  Mux1/1 -> SSN OLTC xfo v2/1(params)
  Fcn/1 -> x/1
  connections:
  CT1/LConn1 -- L/RConn1
  PT/LConn2 -- Ground1/LConn1
  S/RConn1 -- SSN Interface Block (1ph)/LConn1
  SSN OLTC xfo v2/RConn1 -- SSN Interface Block (1ph)2/LConn1
  SSN OLTC xfo v2/LConn1 -- SSN Interface Block (1ph)/RConn1
  PT/LConn1 -- SSN Interface Block (1ph)2/RConn1 -- CT1/RConn1

== system IEEE123_4subsystem/SM_123p/Regulator 2/Single Phase SVR_A/Voltage Regulator Control ==
  Vm : Inport
  Constant : Constant  Value=RegulatorOn
  Tap Changer Control : Subsystem  mask(Tap Changer Control){MinMaxTap=TapMinMax, InitialPosition=InitialTap, MecDelay=TapSelectionTime}
      mask prompts: MinMaxTap "Minimum and maximum tap number [ Min  Max ] :"; InitialPosition "Initial tap position"; MecDelay "Mechanical delay time"
      mask init:
      | if MecDelay<=0,
      | 	MecDelay=1/60;
      | end
  Voltage regulator : Subsystem  mask{Vref=RegulatorVref*120, DeadBand=RegulatorDeadBand*120, TimeDelay=RegulatorDelay}
      mask prompts: Vref "Vref (on 120v base)"; DeadBand "Deadband (on 120v base)"; TimeDelay "Time delay (s)"
  N : Outport
  Tap : Outport  Port=2
  wires:
  Vm/1 -> Voltage regulator/1(Vmes (pu))
  Constant/1 -> Voltage regulator/3(RegOn)
  Tap Changer Control/2(Ready) -> Voltage regulator/2(Ready)
  Voltage regulator/1(Up) -> Tap Changer Control/1("Up ")
  Tap Changer Control/1(TapNo) -> N/1, Tap/1  "Tap"
  Voltage regulator/2(Down) -> Tap Changer Control/2("Down ")

== system IEEE123_4subsystem/SS_123p1/Regulator 4/Single Phase SVR_A/Line Drop Compensator ==
  note: Vm=Vsec-Isec(Rc+jXc)
  Isec : Inport
  Vsec : Inport  Port=2
  "        " : spsLinearTransformerLib/Linear Transformer  UNITS=SI  NominalPower=[pNom fNom]  winding1=[vNom/ptRatio 1e-7 1e-8]  winding2=[vNom/ptRatio 1e-7 1e-8]  ThreeWindings=off  winding3=[3.15e+005 0.7938 0.084225]  RmLm=[1e5 1e5]  Measurements=None  DataType=on
  "CTS  " : spsControlledCurrentSourceLib/Controlled Current Source  Initialize=on  Source_Type=AC  Amplitude=0  Phase=0  Frequency=0  Measurements=None
  "PTS  " : spsControlledVoltageSourceLib/Controlled Voltage Source  Initialize=on  Source_Type=AC  Amplitude=0  Phase=0  Frequency=0  Measurements=None
  RMS : spsRMSLib/RMS  TrueRMS=on  Freq=60  RMSInit=120  Ts=0
  Raux : spsSeriesRLCBranchLib/Series RLC Branch  LConnTagsString=__new0  RConnTagsString=__new0  BranchType=R  Resistance=1e3  Inductance=1.6 / (120*pi)  SetiL0=off  InitialCurrent=0  Capacitance=1e-6  Setx0=off  InitialVoltage=0  Measurements=None
  Rc+jXc : spsSeriesRLCBranchLib/Series RLC Branch  LConnTagsString=__new0  RConnTagsString=__new0  BranchType=RL  Resistance=Rc  Inductance=Xc / (2*pi*fNom)  SetiL0=off  InitialCurrent=0  Capacitance=1e-6  Setx0=off  InitialVoltage=0  Measurements=None
  VRelay : spsVoltageMeasurementLib/Voltage Measurement  PhasorSimulation=off  OutputType=Complex  PSBequivalent=0
  Vm : Outport
  wires:
  RMS/1 -> Vm/1
  VRelay/1 -> RMS/1
  Isec/1 -> "CTS  "/1
  Vsec/1 -> "PTS  "/1
  connections:
  "PTS  "/RConn1 -- "        "/RConn1
  "        "/RConn2 -- VRelay/LConn1
  Raux/LConn1 -- Rc+jXc/LConn1 -- "        "/LConn1 -- "CTS  "/RConn1
  Rc+jXc/RConn1 -- Raux/RConn1 -- "CTS  "/LConn1 -- "        "/LConn2
  VRelay/LConn2 -- "PTS  "/LConn1
